simulink model "Biomodel2ss"  (R2017b)
settings: Solver=VariableStepAuto  StartTime=0.0  StopTime=10.0  RelTol=1e-3
libraries: fl_lib x4
settings Model: Creator=Warsars  LastModifiedBy=Warsars

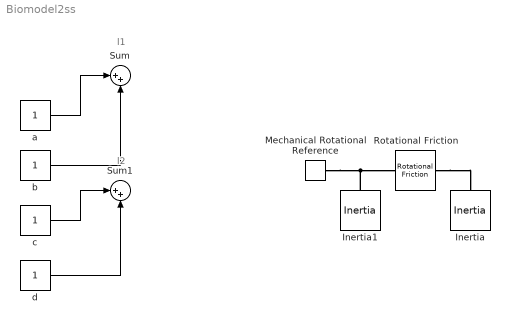
== system Biomodel2ss ==
  note: l2
  note: l1
  Inertia : fl_lib/Mechanical/Rotational Elements/Inertia  inertia=teta2 kg*m^2  w_specify=off  w_priority=High  w=0 rad/s  w_nominal_specify=off  w_nominal_unit=rad/s  w_nominal_value=1  t_specify=off  t_priority=None  t=0 N*m  t_nominal_specify=off  t_nominal_unit=N*m  t_nominal_value=1
  Inertia1 : fl_lib/Mechanical/Rotational Elements/Inertia  inertia=teta1 kg*m^2  w_specify=off  w_priority=High  w=0 rad/s  w_nominal_specify=off  w_nominal_unit=rad/s  w_nominal_value=1  t_specify=off  t_priority=None  t=0 N*m  t_nominal_specify=off  t_nominal_unit=N*m  t_nominal_value=1
  Mechanical Rotational Reference : fl_lib/Mechanical/Rotational Elements/Mechanical Rotational Reference
  Rotational Friction : fl_lib/Mechanical/Rotational Elements/Rotational Friction  brkwy_trq=0 N*m  brkwy_vel=0 rad/s  Col_trq=0 N*m  visc_coef=0 N*m/(rad/s)  w_specify=off  w_priority=None  w=0 rad/s  w_nominal_specify=off  w_nominal_unit=rad/s  w_nominal_value=1  t_specify=off  t_priority=None  t=0 N*m  t_nominal_specify=off  t_nominal_unit=N*m  t_nominal_value=1
      settings: SourceProductName=Simscape
  Sum : Sum  Inputs=|++
  Sum1 : Sum  Inputs=|++
  a : Constant
  b : Constant
  c : Constant
  d : Constant
  wires:
  a/1 -> Sum/1
  b/1 -> Sum/2
  c/1 -> Sum1/1
  d/1 -> Sum1/2
  connections:
  Inertia1/LConn1 -- Rotational Friction/LConn1 -- Mechanical Rotational Reference/LConn1
  Rotational Friction/RConn1 -- Inertia/LConn1
